simulink model "SingleWorkstation_ThreeInParallel"  (R2015a)
settings: Solver=ode45  StartTime=0.0  StopTime=100000  RelTol=1e-3
InitFcn:
  | se_randomizeseeds(gcs, 'Mode', 'All')
undefined symbols (not defined in the file): se_randomizeseeds
libraries: simeventslib x3
settings Model: CovSFcnEnable=off  Creator=gthiers3  LastModifiedBy=AnotherUser
settings DebuggingCC: SolverPrmCheckMsg=warning

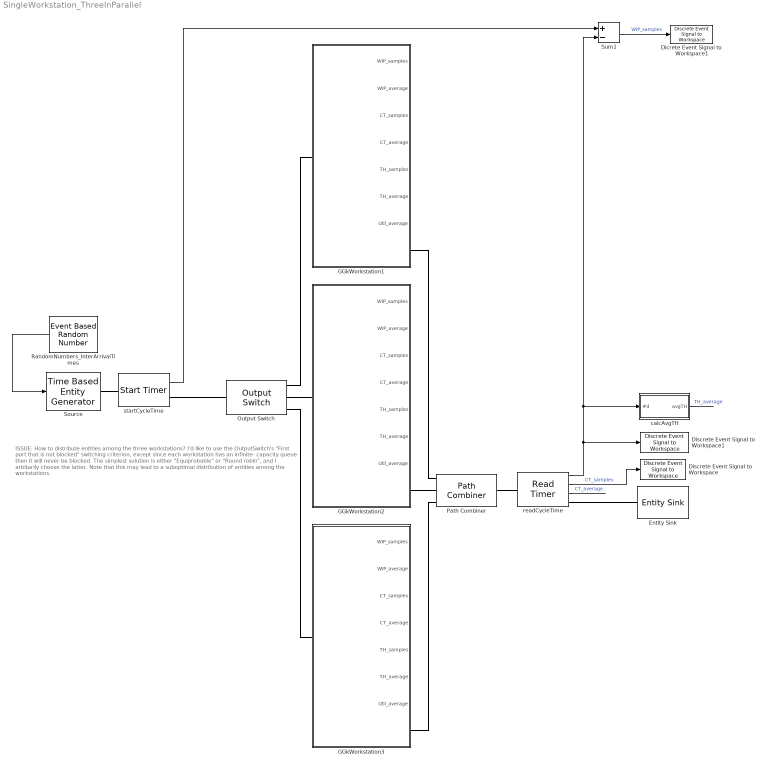
== system SingleWorkstation_ThreeInParallel ==
  note: ISSUE: How to distribute entities among the three workstations?
      |
      | I'd like to use the OutputSwitch's "First port that is not blocked"
      | switching criterion, except since each workstation has an infinite-
      | capacity queue then it will never be blocked.
      |
      | The simplest solution is either "Equiprobable" or "Round robin",
      | and I arbitarily choose the latter. Note that this may lead to a
      | suboptimal distribution of entities among the workstations.
  Dicrete Event Signal to Workspace1 : simeventslib/SimEvents Sinks/Discrete Event Signal to Workspace  VariableName=WIP  SaveFormat=Structure With Time  isMonitorOnly=off  isRecordIC=off
  Discrete Event Signal to Workspace : simeventslib/SimEvents Sinks/Discrete Event Signal to Workspace  VariableName=CycleTime  SaveFormat=Structure With Time  isMonitorOnly=off  isRecordIC=off
  Discrete Event Signal to Workspace1 : simeventslib/SimEvents Sinks/Discrete Event Signal to Workspace  VariableName=Departures  SaveFormat=Structure With Time  isMonitorOnly=off  isRecordIC=off
  Entity Sink : EntitySink
  GGkWorkstation1 : Subsystem  InitFcn=se_randomizeseeds(gcs, 'Mode', 'All')
      settings: CopyFcn=set_param(gcb, 'LinkStatus', 'none');
  GGkWorkstation2 : Subsystem  InitFcn=se_randomizeseeds(gcs, 'Mode', 'All')
      settings: CopyFcn=set_param(gcb, 'LinkStatus', 'none');
  GGkWorkstation3 : Subsystem  InitFcn=se_randomizeseeds(gcs, 'Mode', 'All')
      settings: CopyFcn=set_param(gcb, 'LinkStatus', 'none');
  Output Switch : OutputSwitch  SwitchingCriterion=Equiprobable  InitialSeed=43252
  Path Combiner : PathCombiner
  RandomNumbers_InterArrivalTimes : EventBasedRandomNumber  meanExp=2  scaleGam=10  meanNorm=100  stdNorm=eps  Seed=40035
  Source : TimeBasedEntityGenerator  GenerateEntitiesUpon=Intergeneration time from port t
  Sum1 : Sum  Inputs=+-
  calcAvgTH : Subsystem
  readCycleTime : ReadTimer  TimerTag=CycleTime  StatNumberDeparted=on  StatTimeElapsed=on  StatAverageTimeElapsed=on
      settings: OutputPortMap=o0,o2,o3
  startCycleTime : StartTimer  TimerTag=CycleTime  TimerStartedOption=Restart  StatNumberDeparted=on
  wires:
  RandomNumbers_InterArrivalTimes/1 -> Source/1
  readCycleTime/2 -> Discrete Event Signal to Workspace/1  "CT_samples"
  Sum1/1 -> Dicrete Event Signal to Workspace1/1  "WIP_samples"
  readCycleTime/1 -> calcAvgTH/1(#d), Sum1/2, Discrete Event Signal to Workspace1/1
  readCycleTime/3 -> ?  "CT_average"
  calcAvgTH/1(avgTH) -> ?  "TH_average"
  startCycleTime/1 -> Sum1/1
  connections:
  readCycleTime/RConn1 -- Entity Sink/LConn1
  startCycleTime/LConn1 -- Source/RConn1
  Output Switch/LConn1 -- startCycleTime/RConn1
  Output Switch/RConn2 -- GGkWorkstation2/LConn1
  Output Switch/RConn1 -- GGkWorkstation1/LConn1
  Output Switch/RConn3 -- GGkWorkstation3/LConn1
  Path Combiner/RConn1 -- readCycleTime/LConn1
  GGkWorkstation1/RConn1 -- Path Combiner/LConn1
  GGkWorkstation2/RConn1 -- Path Combiner/LConn2
  GGkWorkstation3/RConn1 -- Path Combiner/LConn3

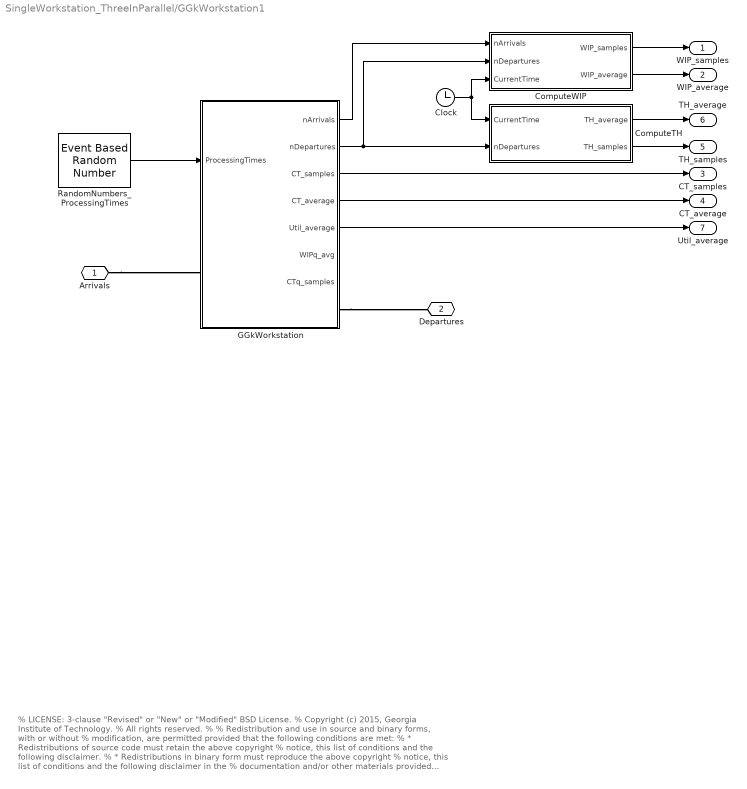
== system SingleWorkstation_ThreeInParallel/GGkWorkstation1 ==
  note: % LICENSE: 3-clause "Revised" or "New" or "Modified" BSD License.
      | % Copyright (c) 2015, Georgia Institute of Technology.
      | % All rights reserved.
      | %
      | % Redistribution and use in source and binary forms, with or without
      | % modification, are permitted provided that the following conditions are met:
      | % * Redistributions of source code must retain the above copyright
      | % notice, this list of conditions and the following disclaimer.
      | % * Redistributions in binary form must reproduce the above copyright
      | % notice, this list of conditions and the following disclaimer in the
      | % documentation and/or other materials provided with the distribution.
      | % * Neither the name of the Georgia Institute of Technology nor the
      | % names of its contributors may be used to endorse or promote products
      | % derived from this software without specific prior written permission.
      | %
      | % THIS SOFTWARE IS PROVIDED BY THE COPYRIGHT HOLDERS AND CONTRIBUTORS "AS IS" AND
      | % ANY EXPRESS OR IMPLIED WARRANTIES, INCLUDING, BUT NOT LIMITED TO, THE IMPLIED
      | % WARRANTIES OF MERCHANTABILITY AND FITNESS FOR A PARTICULAR PURPOSE ARE
      | % DISCLAIMED. IN NO EVENT SHALL THE GEORGIA INSTITUTE OF TECHNOLOGY BE LIABLE FOR
      | % ANY DIRECT, INDIRECT, INCIDENTAL, SPECIAL, EXEMPLARY, OR CONSEQUENTIAL DAMAGES
      | % (INCLUDING, BUT NOT LIMITED TO, PROCUREMENT OF SUBSTITUTE GOODS OR SERVICES;
      | % LOSS OF USE, DATA, OR PROFITS; OR BUSINESS INTERRUPTION) HOWEVER CAUSED AND
      | % ON ANY THEORY OF LIABILITY, WHETHER IN CONTRACT, STRICT LIABILITY, OR TORT
      | % (INCLUDING NEGLIGENCE OR OTHERWISE) ARISING IN ANY WAY OUT OF THE USE OF THIS
      | % SOFTWARE, EVEN IF ADVISED OF THE POSSIBILITY OF SUCH DAMAGE.
  Clock : Clock
  ComputeTH : Subsystem
  ComputeWIP : Subsystem
  GGkWorkstation : Subsystem  mask{Capacity=Inf, NumberOfServers=1}
      mask prompts: Capacity "Queue Capacity:"; NumberOfServers "Number of Servers:"
      mask TypeOptions Capacity: FIFOQueue/Capacity
      mask TypeOptions NumberOfServers: N-Server/NumberOfServers
      mask DialogControl DescTextVar Prompt: Plain-vanilla GGk Workstation, with a FIFOQueue and N-Server
  RandomNumbers_ProcessingTimes : EventBasedRandomNumber  Distribution=Triangular  meanExp=90  minUnif=40  maxUnif=40  pOneBern=40  pSuccessBino=40  numTrialBino=40  maxTri=7  modeTri=4  thresholdGam=40  scaleGam=40  shapeGam=40  meanNorm=95  stdNorm=eps  pSuccessGeo=40  meanPoiss=40  scaleLogn=2.246  shapeLogn=1.395  thresholdLogl=40  scaleLogl=40  minBeta=40  maxBeta=40  shape1Beta=40  shape2Beta=40  minUnid=40  maxUnid=40  numValueUnid=40  thresholdWbl=40  scaleWbl=40  shapeWbl=40  valueVecCont=40  cdfVecCont=40  valueVecDisc=40  probVecDisc=40  Seed=30384
  Arrivals : PMIOPort  Port=1  Side=Left
  Departures : PMIOPort  Port=2  Side=Right
  WIP_samples : Outport
  WIP_average : Outport  Port=2
  CT_samples : Outport  Port=3
  CT_average : Outport  Port=4
  TH_samples : Outport  Port=5
  TH_average : Outport  Port=6
  Util_average : Outport  Port=7
  wires:
  ComputeTH/2(TH_samples) -> TH_samples/1
  ComputeTH/1(TH_average) -> TH_average/1
  Clock/1 -> ComputeTH/1(CurrentTime), ComputeWIP/3(CurrentTime)
  GGkWorkstation/1(nArrivals) -> ComputeWIP/1(nArrivals)
  ComputeWIP/2(WIP_average) -> WIP_average/1
  ComputeWIP/1(WIP_samples) -> WIP_samples/1
  GGkWorkstation/4(CT_average) -> CT_average/1
  GGkWorkstation/3(CT_samples) -> CT_samples/1
  GGkWorkstation/2(nDepartures) -> ComputeWIP/2(nDepartures), ComputeTH/2(nDepartures)
  GGkWorkstation/5(Util_average) -> Util_average/1
  RandomNumbers_ProcessingTimes/1 -> GGkWorkstation/1(ProcessingTimes)
  connections:
  Arrivals/RConn1 -- GGkWorkstation/LConn1
  GGkWorkstation/RConn1 -- Departures/RConn1

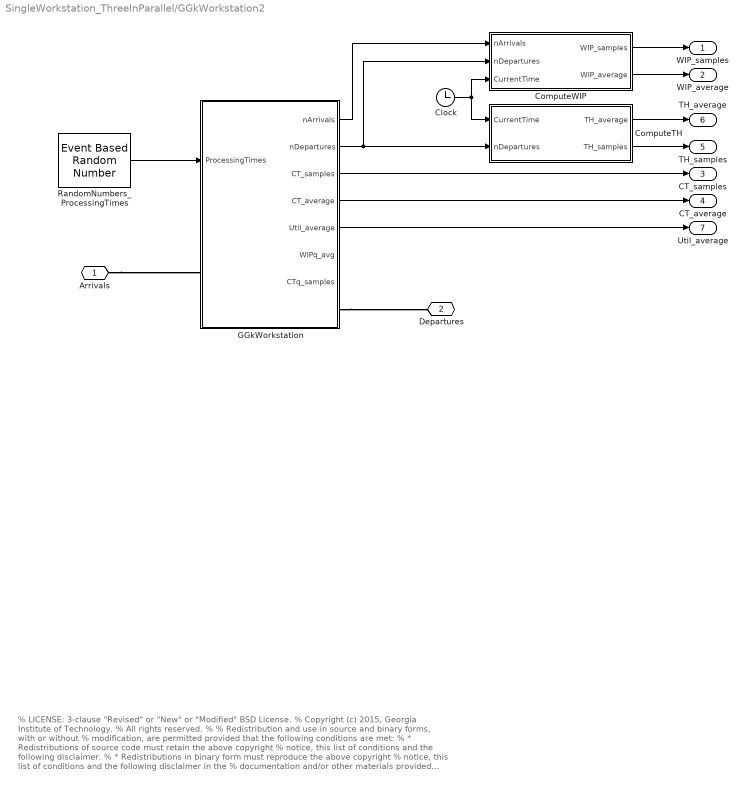
== system SingleWorkstation_ThreeInParallel/GGkWorkstation2 ==
  note: % LICENSE: 3-clause "Revised" or "New" or "Modified" BSD License.
      | % Copyright (c) 2015, Georgia Institute of Technology.
      | % All rights reserved.
      | %
      | % Redistribution and use in source and binary forms, with or without
      | % modification, are permitted provided that the following conditions are met:
      | % * Redistributions of source code must retain the above copyright
      | % notice, this list of conditions and the following disclaimer.
      | % * Redistributions in binary form must reproduce the above copyright
      | % notice, this list of conditions and the following disclaimer in the
      | % documentation and/or other materials provided with the distribution.
      | % * Neither the name of the Georgia Institute of Technology nor the
      | % names of its contributors may be used to endorse or promote products
      | % derived from this software without specific prior written permission.
      | %
      | % THIS SOFTWARE IS PROVIDED BY THE COPYRIGHT HOLDERS AND CONTRIBUTORS "AS IS" AND
      | % ANY EXPRESS OR IMPLIED WARRANTIES, INCLUDING, BUT NOT LIMITED TO, THE IMPLIED
      | % WARRANTIES OF MERCHANTABILITY AND FITNESS FOR A PARTICULAR PURPOSE ARE
      | % DISCLAIMED. IN NO EVENT SHALL THE GEORGIA INSTITUTE OF TECHNOLOGY BE LIABLE FOR
      | % ANY DIRECT, INDIRECT, INCIDENTAL, SPECIAL, EXEMPLARY, OR CONSEQUENTIAL DAMAGES
      | % (INCLUDING, BUT NOT LIMITED TO, PROCUREMENT OF SUBSTITUTE GOODS OR SERVICES;
      | % LOSS OF USE, DATA, OR PROFITS; OR BUSINESS INTERRUPTION) HOWEVER CAUSED AND
      | % ON ANY THEORY OF LIABILITY, WHETHER IN CONTRACT, STRICT LIABILITY, OR TORT
      | % (INCLUDING NEGLIGENCE OR OTHERWISE) ARISING IN ANY WAY OUT OF THE USE OF THIS
      | % SOFTWARE, EVEN IF ADVISED OF THE POSSIBILITY OF SUCH DAMAGE.
  Clock : Clock
  ComputeTH : Subsystem
  ComputeWIP : Subsystem
  GGkWorkstation : Subsystem  mask{Capacity=Inf, NumberOfServers=1}
      mask prompts: Capacity "Queue Capacity:"; NumberOfServers "Number of Servers:"
      mask TypeOptions Capacity: FIFOQueue/Capacity
      mask TypeOptions NumberOfServers: N-Server/NumberOfServers
      mask DialogControl DescTextVar Prompt: Plain-vanilla GGk Workstation, with a FIFOQueue and N-Server
  RandomNumbers_ProcessingTimes : EventBasedRandomNumber  Distribution=Triangular  meanExp=90  minUnif=40  maxUnif=40  pOneBern=40  pSuccessBino=40  numTrialBino=40  maxTri=7  modeTri=4  thresholdGam=40  scaleGam=40  shapeGam=40  meanNorm=95  stdNorm=eps  pSuccessGeo=40  meanPoiss=40  scaleLogn=2.246  shapeLogn=1.395  thresholdLogl=40  scaleLogl=40  minBeta=40  maxBeta=40  shape1Beta=40  shape2Beta=40  minUnid=40  maxUnid=40  numValueUnid=40  thresholdWbl=40  scaleWbl=40  shapeWbl=40  valueVecCont=40  cdfVecCont=40  valueVecDisc=40  probVecDisc=40  Seed=33601
  Arrivals : PMIOPort  Port=1  Side=Left
  Departures : PMIOPort  Port=2  Side=Right
  WIP_samples : Outport
  WIP_average : Outport  Port=2
  CT_samples : Outport  Port=3
  CT_average : Outport  Port=4
  TH_samples : Outport  Port=5
  TH_average : Outport  Port=6
  Util_average : Outport  Port=7
  wires:
  ComputeTH/2(TH_samples) -> TH_samples/1
  ComputeTH/1(TH_average) -> TH_average/1
  Clock/1 -> ComputeTH/1(CurrentTime), ComputeWIP/3(CurrentTime)
  GGkWorkstation/1(nArrivals) -> ComputeWIP/1(nArrivals)
  ComputeWIP/2(WIP_average) -> WIP_average/1
  ComputeWIP/1(WIP_samples) -> WIP_samples/1
  GGkWorkstation/4(CT_average) -> CT_average/1
  GGkWorkstation/3(CT_samples) -> CT_samples/1
  GGkWorkstation/2(nDepartures) -> ComputeWIP/2(nDepartures), ComputeTH/2(nDepartures)
  GGkWorkstation/5(Util_average) -> Util_average/1
  RandomNumbers_ProcessingTimes/1 -> GGkWorkstation/1(ProcessingTimes)
  connections:
  Arrivals/RConn1 -- GGkWorkstation/LConn1
  GGkWorkstation/RConn1 -- Departures/RConn1

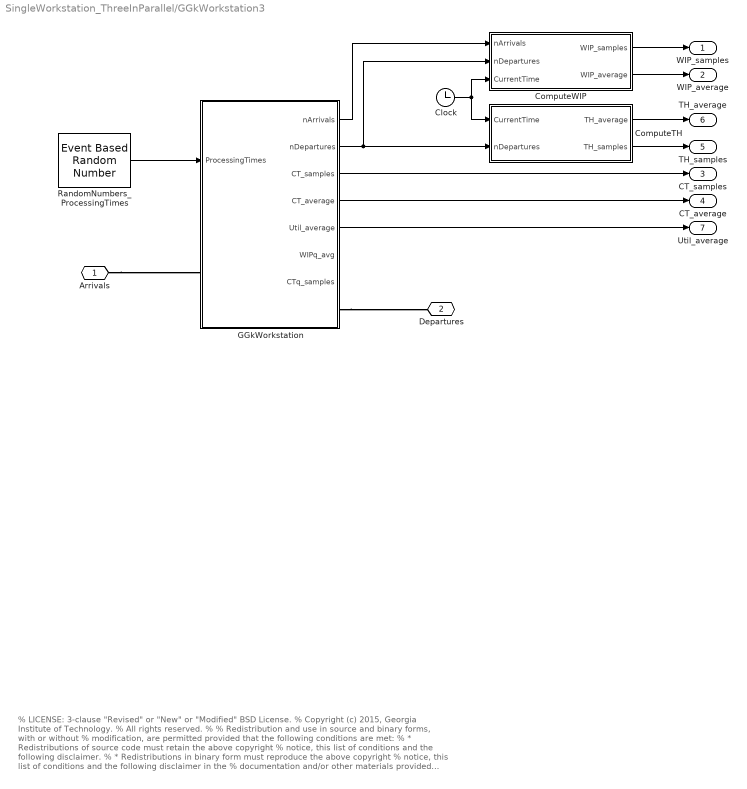
== system SingleWorkstation_ThreeInParallel/GGkWorkstation3 ==
  note: % LICENSE: 3-clause "Revised" or "New" or "Modified" BSD License.
      | % Copyright (c) 2015, Georgia Institute of Technology.
      | % All rights reserved.
      | %
      | % Redistribution and use in source and binary forms, with or without
      | % modification, are permitted provided that the following conditions are met:
      | % * Redistributions of source code must retain the above copyright
      | % notice, this list of conditions and the following disclaimer.
      | % * Redistributions in binary form must reproduce the above copyright
      | % notice, this list of conditions and the following disclaimer in the
      | % documentation and/or other materials provided with the distribution.
      | % * Neither the name of the Georgia Institute of Technology nor the
      | % names of its contributors may be used to endorse or promote products
      | % derived from this software without specific prior written permission.
      | %
      | % THIS SOFTWARE IS PROVIDED BY THE COPYRIGHT HOLDERS AND CONTRIBUTORS "AS IS" AND
      | % ANY EXPRESS OR IMPLIED WARRANTIES, INCLUDING, BUT NOT LIMITED TO, THE IMPLIED
      | % WARRANTIES OF MERCHANTABILITY AND FITNESS FOR A PARTICULAR PURPOSE ARE
      | % DISCLAIMED. IN NO EVENT SHALL THE GEORGIA INSTITUTE OF TECHNOLOGY BE LIABLE FOR
      | % ANY DIRECT, INDIRECT, INCIDENTAL, SPECIAL, EXEMPLARY, OR CONSEQUENTIAL DAMAGES
      | % (INCLUDING, BUT NOT LIMITED TO, PROCUREMENT OF SUBSTITUTE GOODS OR SERVICES;
      | % LOSS OF USE, DATA, OR PROFITS; OR BUSINESS INTERRUPTION) HOWEVER CAUSED AND
      | % ON ANY THEORY OF LIABILITY, WHETHER IN CONTRACT, STRICT LIABILITY, OR TORT
      | % (INCLUDING NEGLIGENCE OR OTHERWISE) ARISING IN ANY WAY OUT OF THE USE OF THIS
      | % SOFTWARE, EVEN IF ADVISED OF THE POSSIBILITY OF SUCH DAMAGE.
  Clock : Clock
  ComputeTH : Subsystem
  ComputeWIP : Subsystem
  GGkWorkstation : Subsystem  mask{Capacity=Inf, NumberOfServers=1}
      mask prompts: Capacity "Queue Capacity:"; NumberOfServers "Number of Servers:"
      mask TypeOptions Capacity: FIFOQueue/Capacity
      mask TypeOptions NumberOfServers: N-Server/NumberOfServers
      mask DialogControl DescTextVar Prompt: Plain-vanilla GGk Workstation, with a FIFOQueue and N-Server
  RandomNumbers_ProcessingTimes : EventBasedRandomNumber  Distribution=Triangular  meanExp=90  minUnif=40  maxUnif=40  pOneBern=40  pSuccessBino=40  numTrialBino=40  maxTri=7  modeTri=4  thresholdGam=40  scaleGam=40  shapeGam=40  meanNorm=95  stdNorm=eps  pSuccessGeo=40  meanPoiss=40  scaleLogn=2.246  shapeLogn=1.395  thresholdLogl=40  scaleLogl=40  minBeta=40  maxBeta=40  shape1Beta=40  shape2Beta=40  minUnid=40  maxUnid=40  numValueUnid=40  thresholdWbl=40  scaleWbl=40  shapeWbl=40  valueVecCont=40  cdfVecCont=40  valueVecDisc=40  probVecDisc=40  Seed=36818
  Arrivals : PMIOPort  Port=1  Side=Left
  Departures : PMIOPort  Port=2  Side=Right
  WIP_samples : Outport
  WIP_average : Outport  Port=2
  CT_samples : Outport  Port=3
  CT_average : Outport  Port=4
  TH_samples : Outport  Port=5
  TH_average : Outport  Port=6
  Util_average : Outport  Port=7
  wires:
  ComputeTH/2(TH_samples) -> TH_samples/1
  ComputeTH/1(TH_average) -> TH_average/1
  Clock/1 -> ComputeTH/1(CurrentTime), ComputeWIP/3(CurrentTime)
  GGkWorkstation/1(nArrivals) -> ComputeWIP/1(nArrivals)
  ComputeWIP/2(WIP_average) -> WIP_average/1
  ComputeWIP/1(WIP_samples) -> WIP_samples/1
  GGkWorkstation/4(CT_average) -> CT_average/1
  GGkWorkstation/3(CT_samples) -> CT_samples/1
  GGkWorkstation/2(nDepartures) -> ComputeWIP/2(nDepartures), ComputeTH/2(nDepartures)
  GGkWorkstation/5(Util_average) -> Util_average/1
  RandomNumbers_ProcessingTimes/1 -> GGkWorkstation/1(ProcessingTimes)
  connections:
  Arrivals/RConn1 -- GGkWorkstation/LConn1
  GGkWorkstation/RConn1 -- Departures/RConn1

== system SingleWorkstation_ThreeInParallel/calcAvgTH ==
  #d : Inport
  Clock : Clock
  Divide : Product  Inputs=*/
  Signal Latch : SignalLatch  ReadMemoryUpon=Write to memory event
      settings: InputPortMap=u0,u2  OutputPortMap=o2
  Timed to Event Signal : TimedToEventSignal
  avgTH : Outport
  wires:
  #d/1 -> Signal Latch/1, Divide/1
  Timed to Event Signal/1 -> Signal Latch/2
  Signal Latch/1 -> Divide/2
  Clock/1 -> Timed to Event Signal/1
  Divide/1 -> avgTH/1

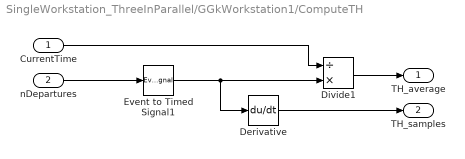
== system SingleWorkstation_ThreeInParallel/GGkWorkstation1/ComputeTH ==
  CurrentTime : Inport
  nDepartures : Inport  Port=2
  Derivative : Derivative
  Divide1 : Product  Inputs=/*
  Event to Timed Signal1 : EventToTimedSignal
  TH_average : Outport
  TH_samples : Outport  Port=2
  wires:
  nDepartures/1 -> Event to Timed Signal1/1
  Derivative/1 -> TH_samples/1
  Divide1/1 -> TH_average/1
  Event to Timed Signal1/1 -> Divide1/2, Derivative/1
  CurrentTime/1 -> Divide1/1

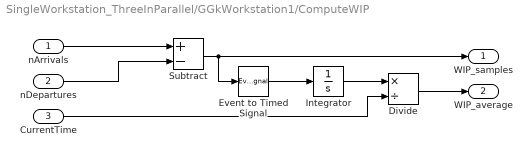
== system SingleWorkstation_ThreeInParallel/GGkWorkstation1/ComputeWIP ==
  nArrivals : Inport
  nDepartures : Inport  Port=2
  CurrentTime : Inport  Port=3
  Divide : Product  Inputs=*/
  Event to Timed Signal : EventToTimedSignal
  Integrator : Integrator
  Subtract : Sum  Inputs=+-
  WIP_samples : Outport
  WIP_average : Outport  Port=2
  wires:
  CurrentTime/1 -> Divide/2
  nDepartures/1 -> Subtract/2
  nArrivals/1 -> Subtract/1
  Integrator/1 -> Divide/1
  Divide/1 -> WIP_average/1
  Event to Timed Signal/1 -> Integrator/1
  Subtract/1 -> Event to Timed Signal/1, WIP_samples/1

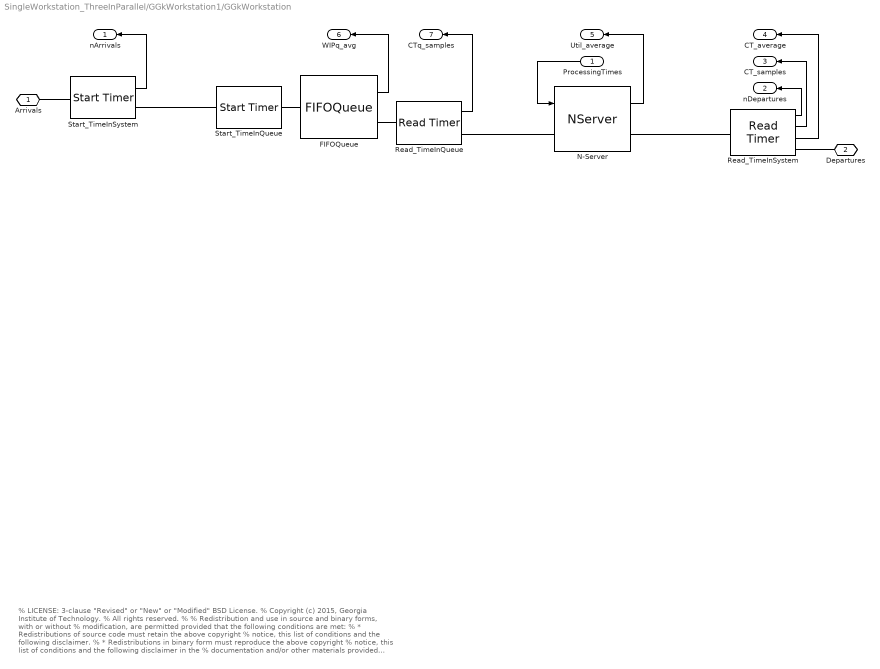
== system SingleWorkstation_ThreeInParallel/GGkWorkstation1/GGkWorkstation ==
  note: % LICENSE: 3-clause "Revised" or "New" or "Modified" BSD License.
      | % Copyright (c) 2015, Georgia Institute of Technology.
      | % All rights reserved.
      | %
      | % Redistribution and use in source and binary forms, with or without
      | % modification, are permitted provided that the following conditions are met:
      | % * Redistributions of source code must retain the above copyright
      | % notice, this list of conditions and the following disclaimer.
      | % * Redistributions in binary form must reproduce the above copyright
      | % notice, this list of conditions and the following disclaimer in the
      | % documentation and/or other materials provided with the distribution.
      | % * Neither the name of the Georgia Institute of Technology nor the
      | % names of its contributors may be used to endorse or promote products
      | % derived from this software without specific prior written permission.
      | %
      | % THIS SOFTWARE IS PROVIDED BY THE COPYRIGHT HOLDERS AND CONTRIBUTORS "AS IS" AND
      | % ANY EXPRESS OR IMPLIED WARRANTIES, INCLUDING, BUT NOT LIMITED TO, THE IMPLIED
      | % WARRANTIES OF MERCHANTABILITY AND FITNESS FOR A PARTICULAR PURPOSE ARE
      | % DISCLAIMED. IN NO EVENT SHALL THE GEORGIA INSTITUTE OF TECHNOLOGY BE LIABLE FOR
      | % ANY DIRECT, INDIRECT, INCIDENTAL, SPECIAL, EXEMPLARY, OR CONSEQUENTIAL DAMAGES
      | % (INCLUDING, BUT NOT LIMITED TO, PROCUREMENT OF SUBSTITUTE GOODS OR SERVICES;
      | % LOSS OF USE, DATA, OR PROFITS; OR BUSINESS INTERRUPTION) HOWEVER CAUSED AND
      | % ON ANY THEORY OF LIABILITY, WHETHER IN CONTRACT, STRICT LIABILITY, OR TORT
      | % (INCLUDING NEGLIGENCE OR OTHERWISE) ARISING IN ANY WAY OUT OF THE USE OF THIS
      | % SOFTWARE, EVEN IF ADVISED OF THE POSSIBILITY OF SUCH DAMAGE.
  ProcessingTimes : Inport
  FIFOQueue : FIFOQueue  Capacity=Capacity  StatAverageQueueLength=on
      settings: OutputPortMap=o3
  N-Server : NServer  NumberOfServers=NumberOfServers  ServiceTimeFrom=Signal port t  StatUtilization=on
      settings: OutputPortMap=o5
  Read_TimeInQueue : ReadTimer  TimerTag=TimeInQueue  StatTimeElapsed=on
      settings: OutputPortMap=o2
  Read_TimeInSystem : ReadTimer  TimerTag=TimeInSystem  StatNumberDeparted=on  StatTimeElapsed=on  StatAverageTimeElapsed=on
      settings: OutputPortMap=o0,o2,o3
  Start_TimeInQueue : StartTimer  TimerTag=TimeInQueue  TimerStartedOption=Restart
  Start_TimeInSystem : StartTimer  TimerTag=TimeInSystem  TimerStartedOption=Restart  StatNumberDeparted=on
  Arrivals : PMIOPort  Port=1  Side=Left
  Departures : PMIOPort  Port=2  Side=Right
  nArrivals : Outport
  nDepartures : Outport  Port=2
  CT_samples : Outport  Port=3
  CT_average : Outport  Port=4
  Util_average : Outport  Port=5
  WIPq_avg : Outport  Port=6
  CTq_samples : Outport  Port=7
  wires:
  Read_TimeInSystem/3 -> CT_average/1
  ProcessingTimes/1 -> N-Server/1
  Read_TimeInSystem/1 -> nDepartures/1
  Start_TimeInSystem/1 -> nArrivals/1
  FIFOQueue/1 -> WIPq_avg/1
  Read_TimeInQueue/1 -> CTq_samples/1
  N-Server/1 -> Util_average/1
  Read_TimeInSystem/2 -> CT_samples/1
  connections:
  Start_TimeInQueue/RConn1 -- FIFOQueue/LConn1
  Read_TimeInQueue/RConn1 -- N-Server/LConn1
  Read_TimeInSystem/RConn1 -- Departures/RConn1
  Start_TimeInSystem/RConn1 -- Start_TimeInQueue/LConn1
  FIFOQueue/RConn1 -- Read_TimeInQueue/LConn1
  N-Server/RConn1 -- Read_TimeInSystem/LConn1
  Arrivals/RConn1 -- Start_TimeInSystem/LConn1

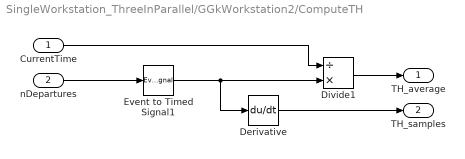
== system SingleWorkstation_ThreeInParallel/GGkWorkstation2/ComputeTH ==
  CurrentTime : Inport
  nDepartures : Inport  Port=2
  Derivative : Derivative
  Divide1 : Product  Inputs=/*
  Event to Timed Signal1 : EventToTimedSignal
  TH_average : Outport
  TH_samples : Outport  Port=2
  wires:
  nDepartures/1 -> Event to Timed Signal1/1
  Derivative/1 -> TH_samples/1
  Divide1/1 -> TH_average/1
  Event to Timed Signal1/1 -> Divide1/2, Derivative/1
  CurrentTime/1 -> Divide1/1

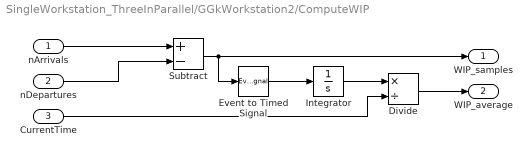
== system SingleWorkstation_ThreeInParallel/GGkWorkstation2/ComputeWIP ==
  nArrivals : Inport
  nDepartures : Inport  Port=2
  CurrentTime : Inport  Port=3
  Divide : Product  Inputs=*/
  Event to Timed Signal : EventToTimedSignal
  Integrator : Integrator
  Subtract : Sum  Inputs=+-
  WIP_samples : Outport
  WIP_average : Outport  Port=2
  wires:
  CurrentTime/1 -> Divide/2
  nDepartures/1 -> Subtract/2
  nArrivals/1 -> Subtract/1
  Integrator/1 -> Divide/1
  Divide/1 -> WIP_average/1
  Event to Timed Signal/1 -> Integrator/1
  Subtract/1 -> Event to Timed Signal/1, WIP_samples/1

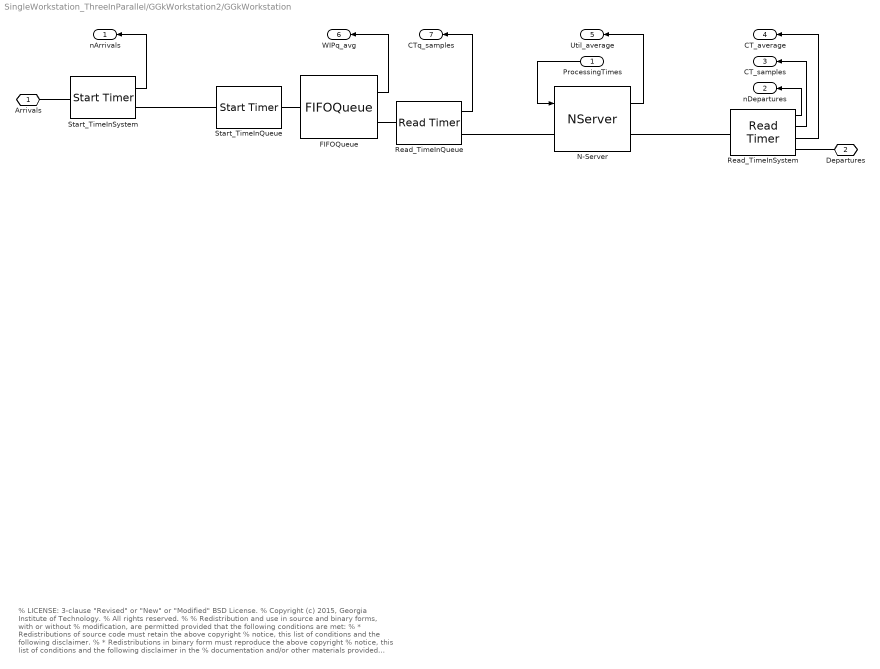
== system SingleWorkstation_ThreeInParallel/GGkWorkstation2/GGkWorkstation ==
  note: % LICENSE: 3-clause "Revised" or "New" or "Modified" BSD License.
      | % Copyright (c) 2015, Georgia Institute of Technology.
      | % All rights reserved.
      | %
      | % Redistribution and use in source and binary forms, with or without
      | % modification, are permitted provided that the following conditions are met:
      | % * Redistributions of source code must retain the above copyright
      | % notice, this list of conditions and the following disclaimer.
      | % * Redistributions in binary form must reproduce the above copyright
      | % notice, this list of conditions and the following disclaimer in the
      | % documentation and/or other materials provided with the distribution.
      | % * Neither the name of the Georgia Institute of Technology nor the
      | % names of its contributors may be used to endorse or promote products
      | % derived from this software without specific prior written permission.
      | %
      | % THIS SOFTWARE IS PROVIDED BY THE COPYRIGHT HOLDERS AND CONTRIBUTORS "AS IS" AND
      | % ANY EXPRESS OR IMPLIED WARRANTIES, INCLUDING, BUT NOT LIMITED TO, THE IMPLIED
      | % WARRANTIES OF MERCHANTABILITY AND FITNESS FOR A PARTICULAR PURPOSE ARE
      | % DISCLAIMED. IN NO EVENT SHALL THE GEORGIA INSTITUTE OF TECHNOLOGY BE LIABLE FOR
      | % ANY DIRECT, INDIRECT, INCIDENTAL, SPECIAL, EXEMPLARY, OR CONSEQUENTIAL DAMAGES
      | % (INCLUDING, BUT NOT LIMITED TO, PROCUREMENT OF SUBSTITUTE GOODS OR SERVICES;
      | % LOSS OF USE, DATA, OR PROFITS; OR BUSINESS INTERRUPTION) HOWEVER CAUSED AND
      | % ON ANY THEORY OF LIABILITY, WHETHER IN CONTRACT, STRICT LIABILITY, OR TORT
      | % (INCLUDING NEGLIGENCE OR OTHERWISE) ARISING IN ANY WAY OUT OF THE USE OF THIS
      | % SOFTWARE, EVEN IF ADVISED OF THE POSSIBILITY OF SUCH DAMAGE.
  ProcessingTimes : Inport
  FIFOQueue : FIFOQueue  Capacity=Capacity  StatAverageQueueLength=on
      settings: OutputPortMap=o3
  N-Server : NServer  NumberOfServers=NumberOfServers  ServiceTimeFrom=Signal port t  StatUtilization=on
      settings: OutputPortMap=o5
  Read_TimeInQueue : ReadTimer  TimerTag=TimeInQueue  StatTimeElapsed=on
      settings: OutputPortMap=o2
  Read_TimeInSystem : ReadTimer  TimerTag=TimeInSystem  StatNumberDeparted=on  StatTimeElapsed=on  StatAverageTimeElapsed=on
      settings: OutputPortMap=o0,o2,o3
  Start_TimeInQueue : StartTimer  TimerTag=TimeInQueue  TimerStartedOption=Restart
  Start_TimeInSystem : StartTimer  TimerTag=TimeInSystem  TimerStartedOption=Restart  StatNumberDeparted=on
  Arrivals : PMIOPort  Port=1  Side=Left
  Departures : PMIOPort  Port=2  Side=Right
  nArrivals : Outport
  nDepartures : Outport  Port=2
  CT_samples : Outport  Port=3
  CT_average : Outport  Port=4
  Util_average : Outport  Port=5
  WIPq_avg : Outport  Port=6
  CTq_samples : Outport  Port=7
  wires:
  Read_TimeInSystem/3 -> CT_average/1
  ProcessingTimes/1 -> N-Server/1
  Read_TimeInSystem/1 -> nDepartures/1
  Start_TimeInSystem/1 -> nArrivals/1
  FIFOQueue/1 -> WIPq_avg/1
  Read_TimeInQueue/1 -> CTq_samples/1
  N-Server/1 -> Util_average/1
  Read_TimeInSystem/2 -> CT_samples/1
  connections:
  Start_TimeInQueue/RConn1 -- FIFOQueue/LConn1
  Read_TimeInQueue/RConn1 -- N-Server/LConn1
  Read_TimeInSystem/RConn1 -- Departures/RConn1
  Start_TimeInSystem/RConn1 -- Start_TimeInQueue/LConn1
  FIFOQueue/RConn1 -- Read_TimeInQueue/LConn1
  N-Server/RConn1 -- Read_TimeInSystem/LConn1
  Arrivals/RConn1 -- Start_TimeInSystem/LConn1

== system SingleWorkstation_ThreeInParallel/GGkWorkstation3/ComputeTH ==
  CurrentTime : Inport
  nDepartures : Inport  Port=2
  Derivative : Derivative
  Divide1 : Product  Inputs=/*
  Event to Timed Signal1 : EventToTimedSignal
  TH_average : Outport
  TH_samples : Outport  Port=2
  wires:
  nDepartures/1 -> Event to Timed Signal1/1
  Derivative/1 -> TH_samples/1
  Divide1/1 -> TH_average/1
  Event to Timed Signal1/1 -> Divide1/2, Derivative/1
  CurrentTime/1 -> Divide1/1

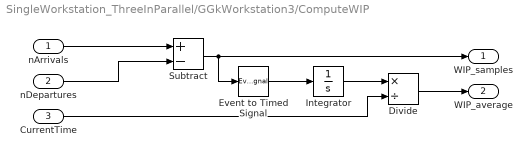
== system SingleWorkstation_ThreeInParallel/GGkWorkstation3/ComputeWIP ==
  nArrivals : Inport
  nDepartures : Inport  Port=2
  CurrentTime : Inport  Port=3
  Divide : Product  Inputs=*/
  Event to Timed Signal : EventToTimedSignal
  Integrator : Integrator
  Subtract : Sum  Inputs=+-
  WIP_samples : Outport
  WIP_average : Outport  Port=2
  wires:
  CurrentTime/1 -> Divide/2
  nDepartures/1 -> Subtract/2
  nArrivals/1 -> Subtract/1
  Integrator/1 -> Divide/1
  Divide/1 -> WIP_average/1
  Event to Timed Signal/1 -> Integrator/1
  Subtract/1 -> Event to Timed Signal/1, WIP_samples/1

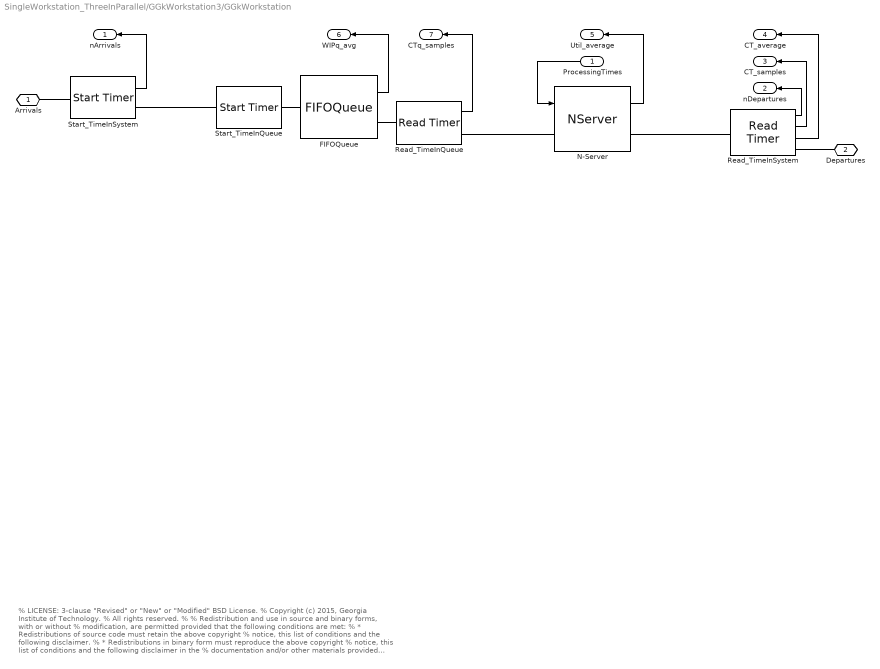
== system SingleWorkstation_ThreeInParallel/GGkWorkstation3/GGkWorkstation ==
  note: % LICENSE: 3-clause "Revised" or "New" or "Modified" BSD License.
      | % Copyright (c) 2015, Georgia Institute of Technology.
      | % All rights reserved.
      | %
      | % Redistribution and use in source and binary forms, with or without
      | % modification, are permitted provided that the following conditions are met:
      | % * Redistributions of source code must retain the above copyright
      | % notice, this list of conditions and the following disclaimer.
      | % * Redistributions in binary form must reproduce the above copyright
      | % notice, this list of conditions and the following disclaimer in the
      | % documentation and/or other materials provided with the distribution.
      | % * Neither the name of the Georgia Institute of Technology nor the
      | % names of its contributors may be used to endorse or promote products
      | % derived from this software without specific prior written permission.
      | %
      | % THIS SOFTWARE IS PROVIDED BY THE COPYRIGHT HOLDERS AND CONTRIBUTORS "AS IS" AND
      | % ANY EXPRESS OR IMPLIED WARRANTIES, INCLUDING, BUT NOT LIMITED TO, THE IMPLIED
      | % WARRANTIES OF MERCHANTABILITY AND FITNESS FOR A PARTICULAR PURPOSE ARE
      | % DISCLAIMED. IN NO EVENT SHALL THE GEORGIA INSTITUTE OF TECHNOLOGY BE LIABLE FOR
      | % ANY DIRECT, INDIRECT, INCIDENTAL, SPECIAL, EXEMPLARY, OR CONSEQUENTIAL DAMAGES
      | % (INCLUDING, BUT NOT LIMITED TO, PROCUREMENT OF SUBSTITUTE GOODS OR SERVICES;
      | % LOSS OF USE, DATA, OR PROFITS; OR BUSINESS INTERRUPTION) HOWEVER CAUSED AND
      | % ON ANY THEORY OF LIABILITY, WHETHER IN CONTRACT, STRICT LIABILITY, OR TORT
      | % (INCLUDING NEGLIGENCE OR OTHERWISE) ARISING IN ANY WAY OUT OF THE USE OF THIS
      | % SOFTWARE, EVEN IF ADVISED OF THE POSSIBILITY OF SUCH DAMAGE.
  ProcessingTimes : Inport
  FIFOQueue : FIFOQueue  Capacity=Capacity  StatAverageQueueLength=on
      settings: OutputPortMap=o3
  N-Server : NServer  NumberOfServers=NumberOfServers  ServiceTimeFrom=Signal port t  StatUtilization=on
      settings: OutputPortMap=o5
  Read_TimeInQueue : ReadTimer  TimerTag=TimeInQueue  StatTimeElapsed=on
      settings: OutputPortMap=o2
  Read_TimeInSystem : ReadTimer  TimerTag=TimeInSystem  StatNumberDeparted=on  StatTimeElapsed=on  StatAverageTimeElapsed=on
      settings: OutputPortMap=o0,o2,o3
  Start_TimeInQueue : StartTimer  TimerTag=TimeInQueue  TimerStartedOption=Restart
  Start_TimeInSystem : StartTimer  TimerTag=TimeInSystem  TimerStartedOption=Restart  StatNumberDeparted=on
  Arrivals : PMIOPort  Port=1  Side=Left
  Departures : PMIOPort  Port=2  Side=Right
  nArrivals : Outport
  nDepartures : Outport  Port=2
  CT_samples : Outport  Port=3
  CT_average : Outport  Port=4
  Util_average : Outport  Port=5
  WIPq_avg : Outport  Port=6
  CTq_samples : Outport  Port=7
  wires:
  Read_TimeInSystem/3 -> CT_average/1
  ProcessingTimes/1 -> N-Server/1
  Read_TimeInSystem/1 -> nDepartures/1
  Start_TimeInSystem/1 -> nArrivals/1
  FIFOQueue/1 -> WIPq_avg/1
  Read_TimeInQueue/1 -> CTq_samples/1
  N-Server/1 -> Util_average/1
  Read_TimeInSystem/2 -> CT_samples/1
  connections:
  Start_TimeInQueue/RConn1 -- FIFOQueue/LConn1
  Read_TimeInQueue/RConn1 -- N-Server/LConn1
  Read_TimeInSystem/RConn1 -- Departures/RConn1
  Start_TimeInSystem/RConn1 -- Start_TimeInQueue/LConn1
  FIFOQueue/RConn1 -- Read_TimeInQueue/LConn1
  N-Server/RConn1 -- Read_TimeInSystem/LConn1
  Arrivals/RConn1 -- Start_TimeInSystem/LConn1
